simulink model "uno"  (R2024a)
settings: Solver=VariableStepAuto  StartTime=0.0  StopTime=20  RelTol=1e-3
settings Model: Creator=ivanc  LastModifiedBy=ivanc

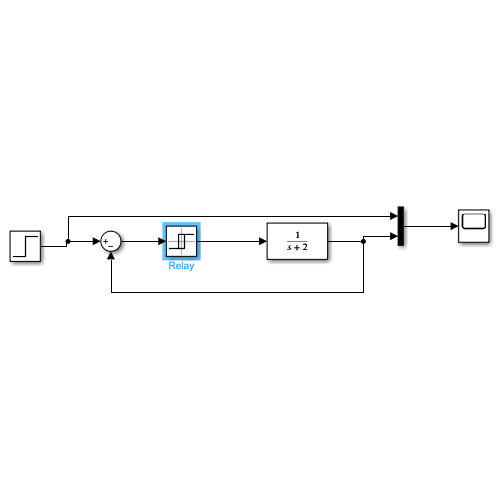
[thumbnail: Simulink's stored preview of the top-level diagram]
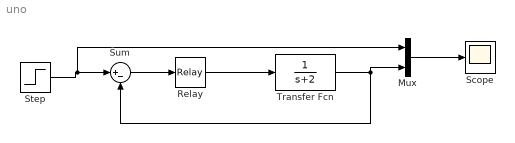
== system uno ==
  Mux : Mux  Inputs=2
  Relay : Relay  OnSwitchValue=0.9  OffSwitchValue=0  OnOutputValue=4  OffOutputValue=2
  Scope : Scope
  Step : Step  Time=10  Before=1  After=2  SampleTime=0
  Sum : Sum  Inputs=|+-
  Transfer Fcn : TransferFcn  Denominator=[1 2]
  wires:
  Mux/1 -> Scope/1
  Transfer Fcn/1 -> Sum/2, Mux/2
  Step/1 -> Mux/1, Sum/1
  Sum/1 -> Relay/1
  Relay/1 -> Transfer Fcn/1
